simulink model "control_model"  (R2015b)
settings: Solver=ode4  StartTime=0.0  StopTime=10  FixedStep=1e-5  RelTol=1e-3
libraries: simulink x4
settings Model: Creator=dkebude  LastModifiedBy=dkebude
settings DataIOCC: ExternalInput=ref  LimitDataPoints=off  LoadExternalInput=on

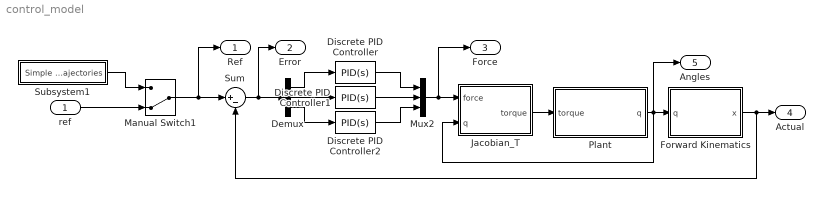
== system control_model ==
  ref : Inport  PortDimensions=3  Interpolate=off
  Demux : Demux  Outputs=3
  Discrete PID Controller : simulink/Continuous/PID Controller  Controller=PID  TimeDomain=Continuous-time  SampleTime=-1  IntegratorMethod=Forward Euler  FilterMethod=Forward Euler  Form=Parallel  UseFilter=on  ControllerParametersSource=internal  P=2776.24169538166  I=81035.833718203  D=23.2241145065613  N=3101.1740850219  InitialConditionSource=internal  InitialConditionForIntegrator=0  InitialConditionForFilter=0  ExternalReset=none  LimitOutput=on  UpperSaturationLimit=1  LowerSaturationLimit=-1  LinearizeAsGain=off  AntiWindupMode=back-calculation  Kb=1  TrackingMode=off  Kt=1  PParamMin=[]  PParamMax=[]  IParamMin=[]  IParamMax=[]  DParamMin=[]  DParamMax=[]  NParamMin=[]  NParamMax=[]  KbParamMin=[]  KbParamMax=[]  KtParamMin=[]  KtParamMax=[]  POutMin=[]  POutMax=[]  IOutMin=[]  IOutMax=[]  DOutMin=[]  DOutMax=[]  NOutMin=[]  NOutMax=[]  KbOutMin=[]  KbOutMax=[]  KtOutMin=[]  KtOutMax=[]  IntegratorOutMin=[]  IntegratorOutMax=[]  FilterOutMin=[]  FilterOutMax=[]  SumOutMin=[]  SumOutMax=[]  SumI1OutMin=[]  SumI1OutMax=[]  SumI2OutMin=[]  SumI2OutMax=[]  SumI3OutMin=[]  SumI3OutMax=[]  SumDOutMin=[]  SumDOutMax=[]  SaturationOutMin=[]  SaturationOutMax=[]  IntegratorContinuousStateAttributes=''  IntegratorStateMustResolveToSignalObject=off  IntegratorRTWStateStorageClass=Auto  FilterContinuousStateAttributes=''  FilterStateMustResolveToSignalObject=off  FilterRTWStateStorageClass=Auto  DifferentiatorICPrevScaledInput=0  DifferentiatorOutMin=[]  DifferentiatorOutMax=[]
  Discrete PID Controller1 : simulink/Continuous/PID Controller  Controller=PID  TimeDomain=Continuous-time  SampleTime=-1  IntegratorMethod=Forward Euler  FilterMethod=Forward Euler  Form=Ideal  UseFilter=on  ControllerParametersSource=internal  P=2704.92783240198  I=31.2046022758799  D=0.00740226480256365  N=1177.16731300035  InitialConditionSource=internal  InitialConditionForIntegrator=0  InitialConditionForFilter=0  ExternalReset=none  LimitOutput=on  UpperSaturationLimit=1  LowerSaturationLimit=-1  LinearizeAsGain=off  AntiWindupMode=none  Kb=1  TrackingMode=off  Kt=1  PParamMin=[]  PParamMax=[]  IParamMin=[]  IParamMax=[]  DParamMin=[]  DParamMax=[]  NParamMin=[]  NParamMax=[]  KbParamMin=[]  KbParamMax=[]  KtParamMin=[]  KtParamMax=[]  POutMin=[]  POutMax=[]  IOutMin=[]  IOutMax=[]  DOutMin=[]  DOutMax=[]  NOutMin=[]  NOutMax=[]  KbOutMin=[]  KbOutMax=[]  KtOutMin=[]  KtOutMax=[]  IntegratorOutMin=[]  IntegratorOutMax=[]  FilterOutMin=[]  FilterOutMax=[]  SumOutMin=[]  SumOutMax=[]  SumI1OutMin=[]  SumI1OutMax=[]  SumI2OutMin=[]  SumI2OutMax=[]  SumI3OutMin=[]  SumI3OutMax=[]  SumDOutMin=[]  SumDOutMax=[]  SaturationOutMin=[]  SaturationOutMax=[]  IntegratorContinuousStateAttributes=''  IntegratorStateMustResolveToSignalObject=off  IntegratorRTWStateStorageClass=Auto  FilterContinuousStateAttributes=''  FilterStateMustResolveToSignalObject=off  FilterRTWStateStorageClass=Auto  DifferentiatorICPrevScaledInput=0  DifferentiatorOutMin=[]  DifferentiatorOutMax=[]
  Discrete PID Controller2 : simulink/Continuous/PID Controller  Controller=PID  TimeDomain=Continuous-time  SampleTime=-1  IntegratorMethod=Forward Euler  FilterMethod=Forward Euler  Form=Parallel  UseFilter=on  ControllerParametersSource=internal  P=8035.43093760868  I=309191.568923046  D=39.2086370141642  N=2821.00025874068  InitialConditionSource=internal  InitialConditionForIntegrator=0  InitialConditionForFilter=0  ExternalReset=none  LimitOutput=on  UpperSaturationLimit=1  LowerSaturationLimit=-1  LinearizeAsGain=off  AntiWindupMode=back-calculation  Kb=1  TrackingMode=off  Kt=1  PParamMin=[]  PParamMax=[]  IParamMin=[]  IParamMax=[]  DParamMin=[]  DParamMax=[]  NParamMin=[]  NParamMax=[]  KbParamMin=[]  KbParamMax=[]  KtParamMin=[]  KtParamMax=[]  POutMin=[]  POutMax=[]  IOutMin=[]  IOutMax=[]  DOutMin=[]  DOutMax=[]  NOutMin=[]  NOutMax=[]  KbOutMin=[]  KbOutMax=[]  KtOutMin=[]  KtOutMax=[]  IntegratorOutMin=[]  IntegratorOutMax=[]  FilterOutMin=[]  FilterOutMax=[]  SumOutMin=[]  SumOutMax=[]  SumI1OutMin=[]  SumI1OutMax=[]  SumI2OutMin=[]  SumI2OutMax=[]  SumI3OutMin=[]  SumI3OutMax=[]  SumDOutMin=[]  SumDOutMax=[]  SaturationOutMin=[]  SaturationOutMax=[]  IntegratorContinuousStateAttributes=''  IntegratorStateMustResolveToSignalObject=off  IntegratorRTWStateStorageClass=Auto  FilterContinuousStateAttributes=''  FilterStateMustResolveToSignalObject=off  FilterRTWStateStorageClass=Auto  DifferentiatorICPrevScaledInput=0  DifferentiatorOutMin=[]  DifferentiatorOutMax=[]
  Forward Kinematics : MATLAB Function  TreatAsAtomicUnit=on
  Jacobian_T : MATLAB Function  TreatAsAtomicUnit=on
  Manual Switch1 : ManualSwitch  CurrentSetting=0
  Mux2 : Mux  Inputs=3
  Plant : Subsystem
  Subsystem1 : Subsystem
  Sum : Sum  Inputs=|+-
  Ref : Outport
  Error : Outport  Port=2
  Force : Outport  Port=3
  Actual : Outport  Port=4
  Angles : Outport  Port=5
  wires:
  Discrete PID Controller/1 -> Mux2/1
  Discrete PID Controller1/1 -> Mux2/2
  Discrete PID Controller2/1 -> Mux2/3
  Mux2/1 -> Force/1, Jacobian_T/1(force)
  Sum/1 -> Error/1, Demux/1
  Demux/1 -> Discrete PID Controller/1
  Demux/2 -> Discrete PID Controller1/1
  Demux/3 -> Discrete PID Controller2/1
  Jacobian_T/1(torque) -> Plant/1(torque)
  Plant/1(q) -> Angles/1, Jacobian_T/2(q), Forward Kinematics/1(q)
  Forward Kinematics/1(x) -> Actual/1, Sum/2
  Manual Switch1/1 -> Ref/1, Sum/1
  Subsystem1/1(Simple Trajectories) -> Manual Switch1/1
  ref/1 -> Manual Switch1/2

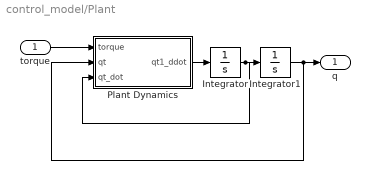
== system control_model/Plant ==
  torque : Inport
  Integrator : Integrator  InitialCondition=[0.0; 0.0; 0.0]
  Integrator1 : Integrator  InitialCondition=[0.0; 0.0; 0.0]
  Plant Dynamics : MATLAB Function  TreatAsAtomicUnit=on
  q : Outport
  wires:
  torque/1 -> Plant Dynamics/1(torque)
  Plant Dynamics/1(qt1_ddot) -> Integrator/1
  Integrator1/1 -> Plant Dynamics/2(qt), q/1
  Integrator/1 -> Plant Dynamics/3(qt_dot), Integrator1/1

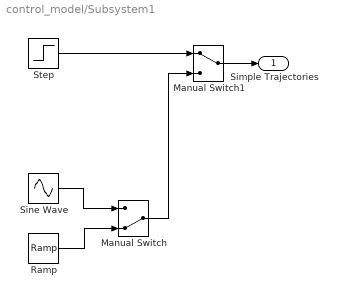
== system control_model/Subsystem1 ==
  Manual Switch : ManualSwitch  CurrentSetting=0
  Manual Switch1 : ManualSwitch
  Ramp : simulink/Sources/Ramp  slope=[0.01; 0.01; 0.01]  start=0  X0=0  VectorParams1D=off
  Sine Wave : Sin  SineType=Sample based  Amplitude=[0.01; 0.01; 0.01]  Phase=[0; pi/8; pi/4]  Samples=1e5  SampleTime=1e-5  VectorParams1D=off
  Step : Step  Before=[0; 0.; 0.]  After=[0.001; 0.001; 0.001]  SampleTime=0  VectorParams1D=off
  Simple Trajectories : Outport
  wires:
  Manual Switch/1 -> Manual Switch1/2
  Manual Switch1/1 -> Simple Trajectories/1
  Ramp/1 -> Manual Switch/2
  Sine Wave/1 -> Manual Switch/1
  Step/1 -> Manual Switch1/1

== matlab function control_model/Forward Kinematics ==
  data: q input; x output
function x = fcn(q)
%#codegen

q1 = q(1); q2 = q(2); q3 = q(3);
l1 = 0.215;%new
l2 = 0.170;

x1 = sin(q1)*(l1*cos(q2)+l2*sin(q3));
x2 = l2 - l2*cos(q3) + l1*sin(q2);
x3 = -l1 + cos(q1)*(l1*cos(q2)+l2*sin(q3));

x = [x1; x2; x3];

== matlab function control_model/Plant/Plant Dynamics ==
  data: torque input; qt1_ddot output; qt input; qt_dot input
function qt1_ddot = fcn(torque, qt, qt_dot)
%#codegen

q1 = qt(1); q2 = qt(2); q3 = qt(3); 
q1d = qt_dot(1); q2d = qt_dot(2); q3d = qt_dot(3); 

%% phantom premium 1.5 parameters
ma = 0.0202;%new
mc = 0.0249;%new
mbe = 0.2359;%new
mdf = 0.1906;
l1 = 0.215;%new
l2 = 0.170;
l3 = 0.0325;
l5 = -36.8e-3;
l6 = 52.7e-3;
g = 9.81;

%% moment of inertia params
Iaxx = 0.4864e-4;
Iayy = 0.001843e-4;
Iazz = 0.4864e-4;
Icxx = 0.959e-4;
Icyy = 0.959e-4;
Iczz = 0.0051e-4;
Ibexx = 11.09e-4;
Ibeyy = 10.06e-4;
Ibezz = 0.591e-4;
Idfxx = 7.11e-4;
Idfyy = 0.629e-4;
Idfzz = 6.246e-4;
Ibaseyy = 11.87e-4;

%% mass matrix components
m11 = (0.125*(4*Iayy+4*Iazz+8*Ibaseyy+4*Ibeyy+4*Ibezz+4*Icyy+4*Iczz+4*Idfyy+4*Idfzz+4*l1*l1*ma+l2*l2*ma+l1*l1*mc+4*l3*l3*mc)...
    +0.125*(4*Ibeyy-4*Ibezz+4*Icyy-4*Iczz+l1*l1*(4*ma+mc))*cos(2*q2)...
    +0.125*(4*Iayy-4*Iazz+4*Idfyy-4*Idfzz-l2*l2*ma-4*l3*l3*mc)*cos(2*q3)+l1*(l2*ma+l3*mc)*cos(q2)*sin(q3));
m22 = 0.25*(4*(Ibexx+Icxx+l1*l1*ma)+l1*l1*mc);
m23 = -0.5*l1*(l2*ma+l3*mc)*sin(q2-q3);
m32 = m23;
m33 = 0.25*(4*Iaxx+4*Idfxx+l2*l2*ma+4*l3*l3*mc);

M = [m11 0 0;
    0 m22 m23;
    0 m32 m33];


%% coriolis matrix components
c11 = 0.125*(-2*sin(q2)*((4*Ibeyy-4*Ibezz+4*Icyy-4*Iczz+4*l1*l1*ma+l1*l1*mc)*cos(q2)+2*l1*(l2*ma+l3*mc)*sin(q3))*q2d...
    +2*cos(q3)*(2*l1*(l2*ma+l3*mc)*cos(q2)+(-4*Iayy+4*Iazz-4*Idfyy+4*Idfzz+l2*l2*ma+4*l3*l3*mc)*sin(q3))*q3d);
c12 = -0.125*((4*Ibeyy-4*Ibezz+4*Icyy-4*Iczz+l1*l1*(4*ma+mc))*sin(2*q2)+4*l1*(l2*ma+l3*mc)*sin(q2)*sin(q3))*q1d;
c13 = -0.125*(-4*l1*(l2*ma+l3*mc)*cos(q2)*cos(q3)-(-4*Iayy+4*Iazz-4*Idfyy+4*Idfzz+l2*l2*ma+4*l3*l3*mc)*sin(2*q3))*q1d;
c21 = -c12;
c22 = 0;
c23 = 0.5*l1*(l2*ma+l3*mc)*cos(q2-q3)*q3d;
c31 = -c13;
c32 = 0.5*l1*(l2*ma+l3*mc)*cos(q2-q3)*q2d;
c33 = 0;

C = [c11 c12 c13;
    c21 c22 c23;
    c31 c32 c33];

%% gravity vector components
tg1 = 0;
tg2 = g*(l1*(ma+0.5*mc)+l5*mbe)*cos(q2);
tg3 = g*(0.5*l2*ma+l3*mc-l6*mdf)*sin(q3);


G = [tg1;
    tg2;
    tg3];

qt1_ddot = M\(torque - C*qt_dot - G);

== matlab function control_model/Jacobian_T ==
  data: force input; q input; torque output
function torque = fcn(force, q)
%#codegen

q1 = q(1); q2 = q(2); q3 = q(3);
l1 = 0.215;%new
l2 = 0.170;

J11 = cos(q1)*(l1*cos(q2)+l2*sin(q3));
J12 = -l1*sin(q1)*sin(q2);
J13 = l2*sin(q1)*cos(q3);
J21 = 0;
J22 = l1*cos(q2);
J23 = l2*sin(q3);
J31 = -sin(q1)*(l1*cos(q2)+l2*sin(q3));
J32 = -l1*cos(q1)*sin(q2);
J33 = l2*cos(q1)*cos(q3);

J = [J11, J12, J13; J21, J22, J23; J31, J32, J33];

torque = J'*force;
